simulink model "FBNREL_Ex05"  (Simulink 10.1)
settings: Solver=ode4  StartTime=0.0  StopTime=inf  FixedStep=dt  RelTol=1e-3  EnableMultiTasking=on
undefined symbols (not defined in the file or in its folder): Parameter
libraries: simulink x1
settings Model: Creator=ivohoutzager  LastModifiedBy=109813  ParamWorkspaceSource=ReferencedWorkspace
settings DataIOCC: LimitDataPoints=on  SaveOutput=off  SignalLogging=off  SaveTime=off
settings OptimizationCC: DefaultParameterBehavior=Inlined  ExpressionDepthLimit=2147483647
settings DebuggingCC: SolverPrmCheckMsg=warning  InheritedTsInSrcMsg=none  FcnCallInpInsideContextMsg=warning  AllowSymbolicDim=off  StateNameClashWarn=warning
settings RTWCC: Description=Bladed Style DLL  SystemTargetFile=discon_grt.tlc  TemplateMakefile=discon_vc_05.tmf  TargetLang=C++  RTWCompilerOptimization=on
settings RTWCC: CustomSource=|
  | Helpers.cpp
  | ExternalParameters.cpp
  | LegacyExternalControllerApi.cpp
settings CodeAppCC: MaxIdLength=63
settings GRTTargetCC: CombineOutputUpdateFcns=on  GRTInterface=off  UseToolchainInfoCompliant=off

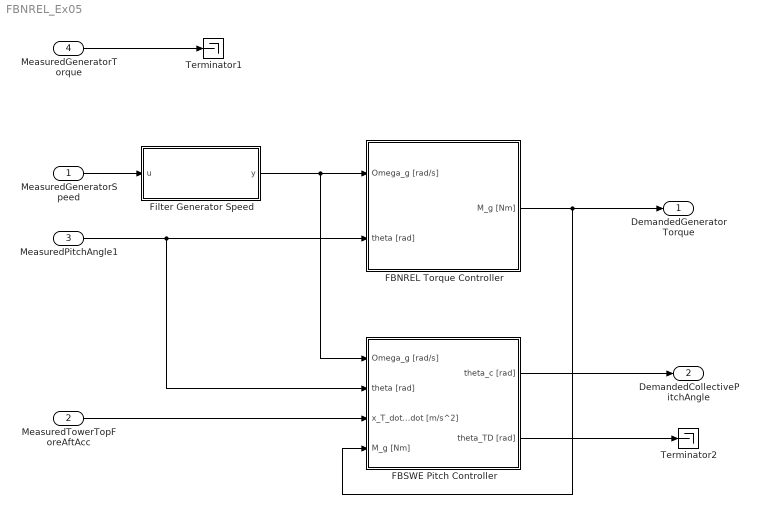
== system FBNREL_Ex05 ==
  MeasuredGeneratorSpeed : Inport  PortDimensions=1
  MeasuredTowerTopForeAftAcc : Inport  Port=2  PortDimensions=1
  MeasuredPitchAngle1 : Inport  Port=3  PortDimensions=1
  MeasuredGeneratorTorque : Inport  Port=4  PortDimensions=1
  FBNREL Torque Controller : Subsystem
  FBSWE Pitch Controller : Subsystem
  Filter Generator Speed : Subsystem
  Terminator1 : Terminator
  Terminator2 : Terminator
  DemandedGeneratorTorque : Outport  PortDimensions=1
  DemandedCollectivePitchAngle : Outport  Port=2  PortDimensions=1
  wires:
  MeasuredGeneratorTorque/1 -> Terminator1/1
  FBNREL Torque Controller/1(M_g [Nm]) -> FBSWE Pitch Controller/4(M_g [Nm]), DemandedGeneratorTorque/1
  MeasuredPitchAngle1/1 -> FBSWE Pitch Controller/2(theta [rad]), FBNREL Torque Controller/2(theta [rad])
  MeasuredGeneratorSpeed/1 -> Filter Generator Speed/1(u)
  Filter Generator Speed/1(y) -> FBSWE Pitch Controller/1(Omega_g [rad/s]), FBNREL Torque Controller/1(Omega_g [rad/s])
  FBSWE Pitch Controller/1(theta_c [rad]) -> DemandedCollectivePitchAngle/1
  FBSWE Pitch Controller/2(theta_TD [rad]) -> Terminator2/1
  MeasuredTowerTopForeAftAcc/1 -> FBSWE Pitch Controller/3(x_T_dotdot [m/s^2])

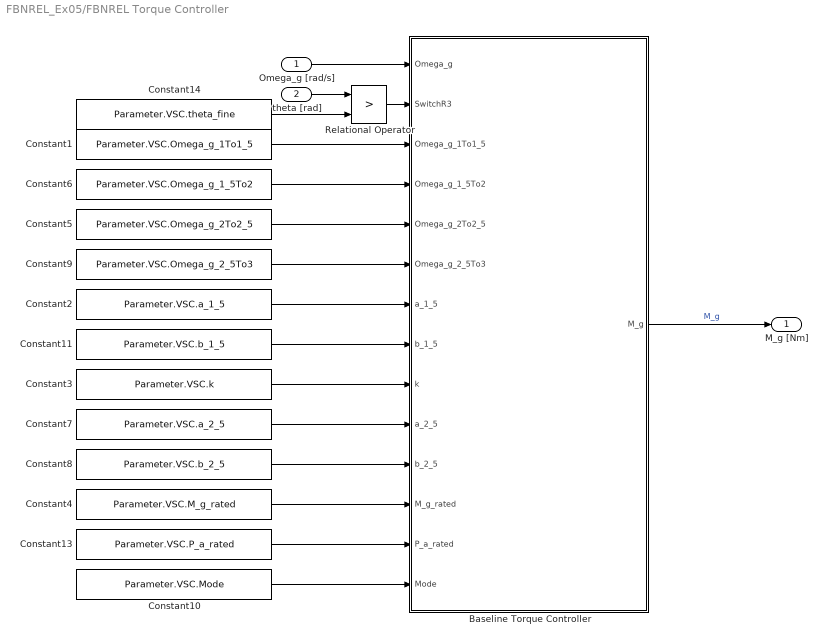
== system FBNREL_Ex05/FBNREL Torque Controller ==
  Omega_g [rad/s] : Inport
  theta [rad] : Inport  Port=2
  Baseline Torque Controller : MATLAB Function  TreatAsAtomicUnit=on
  Constant1 : Constant  Value=Parameter.VSC.Omega_g_1To1_5
  Constant10 : Constant  Value=Parameter.VSC.Mode
  Constant11 : Constant  Value=Parameter.VSC.b_1_5
  Constant13 : Constant  Value=Parameter.VSC.P_a_rated
  Constant14 : Constant  Value=Parameter.VSC.theta_fine
  Constant2 : Constant  Value=Parameter.VSC.a_1_5
  Constant3 : Constant  Value=Parameter.VSC.k
  Constant4 : Constant  Value=Parameter.VSC.M_g_rated
  Constant5 : Constant  Value=Parameter.VSC.Omega_g_2To2_5
  Constant6 : Constant  Value=Parameter.VSC.Omega_g_1_5To2
  Constant7 : Constant  Value=Parameter.VSC.a_2_5
  Constant8 : Constant  Value=Parameter.VSC.b_2_5
  Constant9 : Constant  Value=Parameter.VSC.Omega_g_2_5To3
  Relational Operator : RelationalOperator  Operator=>  OutDataTypeStr=boolean  RndMeth=Nearest
  M_g [Nm] : Outport
  wires:
  Constant13/1 -> Baseline Torque Controller/13(P_a_rated)
  Constant11/1 -> Baseline Torque Controller/8(b_1_5)
  Constant2/1 -> Baseline Torque Controller/7(a_1_5)
  Constant10/1 -> Baseline Torque Controller/14(Mode)
  Constant3/1 -> Baseline Torque Controller/9(k)
  Constant7/1 -> Baseline Torque Controller/10(a_2_5)
  Constant8/1 -> Baseline Torque Controller/11(b_2_5)
  Constant4/1 -> Baseline Torque Controller/12(M_g_rated)
  Constant9/1 -> Baseline Torque Controller/6(Omega_g_2_5To3)
  Constant6/1 -> Baseline Torque Controller/4(Omega_g_1_5To2)
  Constant5/1 -> Baseline Torque Controller/5(Omega_g_2To2_5)
  Constant1/1 -> Baseline Torque Controller/3(Omega_g_1To1_5)
  Baseline Torque Controller/1(M_g) -> M_g [Nm]/1  "M_g"
  Omega_g [rad/s]/1 -> Baseline Torque Controller/1(Omega_g)
  Constant14/1 -> Relational Operator/2
  theta [rad]/1 -> Relational Operator/1
  Relational Operator/1 -> Baseline Torque Controller/2(SwitchR3)

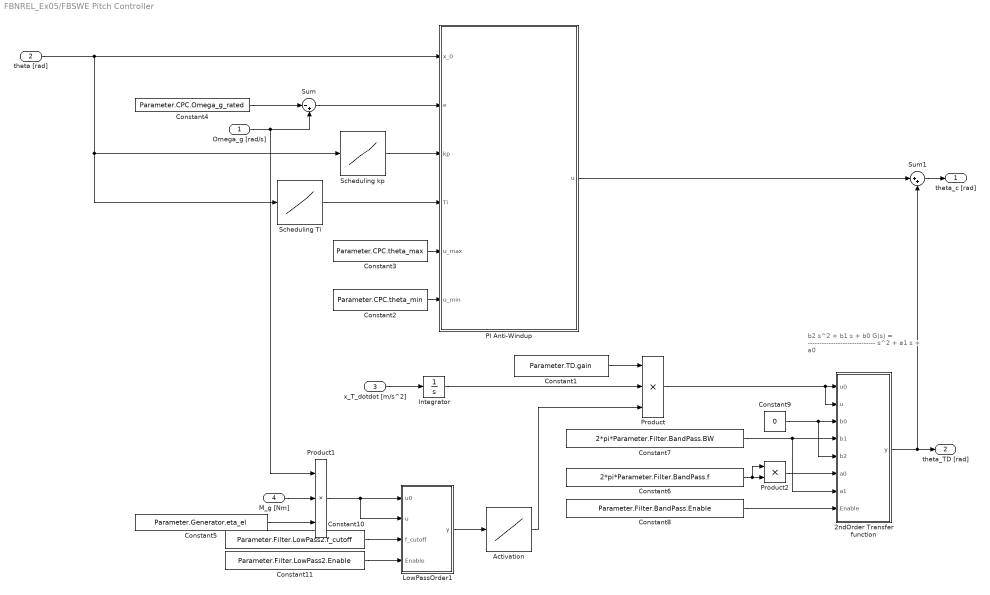
== system FBNREL_Ex05/FBSWE Pitch Controller ==
  note: b2 s^2 + b1 s + b0
      | G(s) = -----------------------------
      | s^2 + a1 s + a0
  Omega_g [rad/s] : Inport
  theta [rad] : Inport  Port=2
  x_T_dotdot [m/s^2] : Inport  Port=3
  M_g [Nm] : Inport  Port=4
  2ndOrder Transfer function : Subsystem
  Activation : Lookup_n-D  NumberOfTableDimensions=1  BreakpointsForDimension1=Parameter.TD.Power  IndexSearchMethod=Linear search  Table=Parameter.TD.Value  ExtrapMethod=Clip  UseLastTableValue=on  InternalRulePriority=Speed  RndMeth=Simplest  InputSameDT=on
  Constant1 : Constant  Value=Parameter.TD.gain
  Constant10 : Constant  Value=Parameter.Filter.LowPass2.f_cutoff
  Constant11 : Constant  Value=Parameter.Filter.LowPass2.Enable
  Constant2 : Constant  Value=Parameter.CPC.theta_min
  Constant3 : Constant  Value=Parameter.CPC.theta_max
  Constant4 : Constant  Value=Parameter.CPC.Omega_g_rated
  Constant5 : Constant  Value=Parameter.Generator.eta_el
  Constant6 : Constant  Value=2*pi*Parameter.Filter.BandPass.f
  Constant7 : Constant  Value=2*pi*Parameter.Filter.BandPass.BW
  Constant8 : Constant  Value=Parameter.Filter.BandPass.Enable
  Constant9 : Constant  Value=0
  Integrator : Integrator
  LowPassOrder1 : Subsystem
  PI Anti-Windup : Subsystem
  Product : Product  Inputs=3
  Product1 : Product  Inputs=***  RndMeth=Zero
  Product2 : Product  RndMeth=Zero
  Scheduling Ti : Lookup_n-D  NumberOfTableDimensions=1  BreakpointsForDimension1=Parameter.CPC.GS.theta  IndexSearchMethod=Linear search  Table=Parameter.CPC.GS.Ti  ExtrapMethod=Clip  UseLastTableValue=on  InternalRulePriority=Speed  RndMeth=Simplest  InputSameDT=on
  Scheduling kp : Lookup_n-D  NumberOfTableDimensions=1  BreakpointsForDimension1=Parameter.CPC.GS.theta  IndexSearchMethod=Linear search  Table=Parameter.CPC.GS.kp  ExtrapMethod=Clip  UseLastTableValue=on  InternalRulePriority=Speed  RndMeth=Simplest  InputSameDT=on
  Sum : Sum  Inputs=|-+
  Sum1 : Sum  Inputs=|++
  theta_c [rad] : Outport
  theta_TD [rad] : Outport  Port=2
  wires:
  Scheduling Ti/1 -> PI Anti-Windup/4(Ti)
  Scheduling kp/1 -> PI Anti-Windup/3(kp)
  theta [rad]/1 -> PI Anti-Windup/1(x_0), Scheduling kp/1, Scheduling Ti/1
  Omega_g [rad/s]/1 -> Product1/1, Sum/2
  Sum/1 -> PI Anti-Windup/2(e)
  Constant2/1 -> PI Anti-Windup/6(u_min)
  Constant3/1 -> PI Anti-Windup/5(u_max)
  Constant4/1 -> Sum/1
  PI Anti-Windup/1(u) -> Sum1/1
  Sum1/1 -> theta_c [rad]/1
  x_T_dotdot [m/s^2]/1 -> Integrator/1
  Integrator/1 -> Product/2
  Constant1/1 -> Product/1
  Activation/1 -> Product/3
  Product/1 -> 2ndOrder Transfer function/2(u), 2ndOrder Transfer function/1(u0)
  Constant8/1 -> 2ndOrder Transfer function/8(Enable)
  Product2/1 -> 2ndOrder Transfer function/6(a0)
  Constant6/1 -> Product2/1, Product2/2
  Constant7/1 -> 2ndOrder Transfer function/7(a1), 2ndOrder Transfer function/4(b1)
  Constant9/1 -> 2ndOrder Transfer function/5(b2), 2ndOrder Transfer function/3(b0)
  Product1/1 -> LowPassOrder1/2(u), LowPassOrder1/1(u0)
  Constant11/1 -> LowPassOrder1/4(Enable)
  Constant10/1 -> LowPassOrder1/3(f_cutoff)
  LowPassOrder1/1(y) -> Activation/1
  M_g [Nm]/1 -> Product1/2
  Constant5/1 -> Product1/3
  2ndOrder Transfer function/1(y) -> theta_TD [rad]/1, Sum1/2

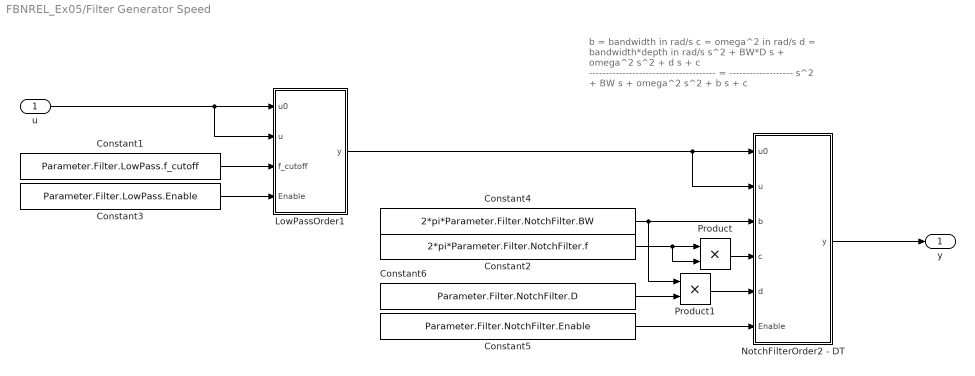
== system FBNREL_Ex05/Filter Generator Speed ==
  note: b = bandwidth in rad/s
      | c = omega^2 in rad/s
      | d = bandwidth*depth in rad/s
      |
      | s^2 + BW*D s + omega^2 s^2 + d s + c
      | -------------------------------------- = -------------------
      | s^2 + BW s + omega^2 s^2 + b s + c
  u : Inport
  Constant1 : Constant  Value=Parameter.Filter.LowPass.f_cutoff
  Constant2 : Constant  Value=2*pi*Parameter.Filter.NotchFilter.f
  Constant3 : Constant  Value=Parameter.Filter.LowPass.Enable
  Constant4 : Constant  Value=2*pi*Parameter.Filter.NotchFilter.BW
  Constant5 : Constant  Value=Parameter.Filter.NotchFilter.Enable
  Constant6 : Constant  Value=Parameter.Filter.NotchFilter.D
  LowPassOrder1 : Subsystem
  NotchFilterOrder2 - DT : Subsystem
  Product : Product  RndMeth=Zero
  Product1 : Product  RndMeth=Zero
  y : Outport
  wires:
  u/1 -> LowPassOrder1/2(u), LowPassOrder1/1(u0)
  Constant3/1 -> LowPassOrder1/4(Enable)
  Constant1/1 -> LowPassOrder1/3(f_cutoff)
  LowPassOrder1/1(y) -> NotchFilterOrder2 - DT/1(u0), NotchFilterOrder2 - DT/2(u)
  Constant5/1 -> NotchFilterOrder2 - DT/6(Enable)
  Product/1 -> NotchFilterOrder2 - DT/4(c)
  Constant2/1 -> Product/2, Product/1
  Constant4/1 -> NotchFilterOrder2 - DT/3(b), Product1/1
  Product1/1 -> NotchFilterOrder2 - DT/5(d)
  Constant6/1 -> Product1/2
  NotchFilterOrder2 - DT/1(y) -> y/1

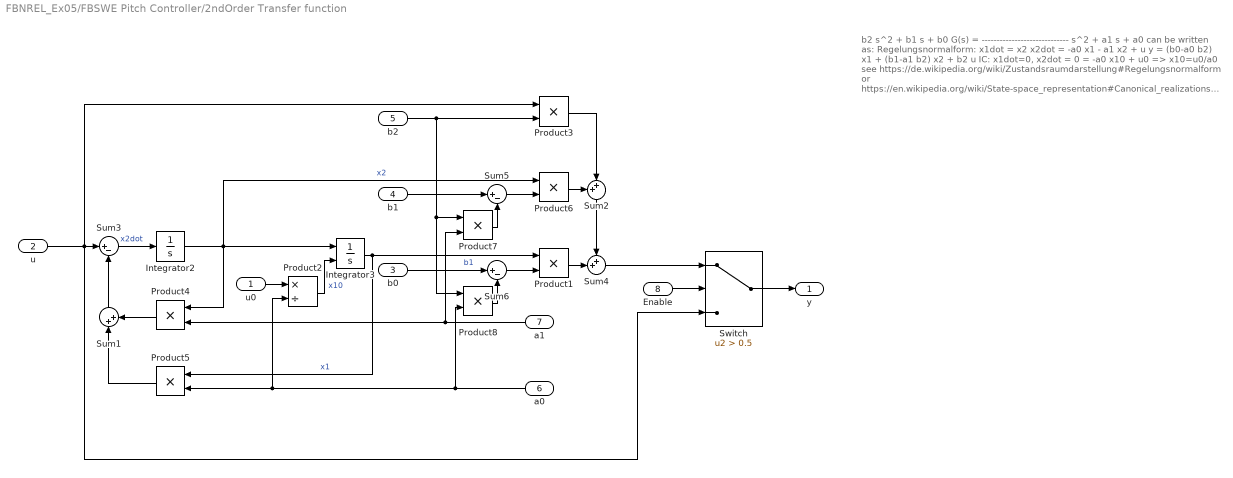
== system FBNREL_Ex05/FBSWE Pitch Controller/2ndOrder Transfer function ==
  note: b2 s^2 + b1 s + b0
      | G(s) = -----------------------------
      | s^2 + a1 s + a0
      |
      | can be written as:
      |
      | Regelungsnormalform:
      | x1dot = x2
      | x2dot = -a0 x1 - a1 x2 + u
      | y = (b0-a0 b2) x1 + (b1-a1 b2) x2 + b2 u
      |
      | IC: x1dot=0, x2dot = 0 = -a0 x10 + u0 => x10=u0/a0
      |
      | see https://de.wikipedia.org/wiki/Zustandsraumdarstellung#Regelungsnormalform
      | or
      | https://en.wikipedia.org/wiki/State-space_representation#Canonical_realizations
      |
      | Advantage:
      | - IC can be set
      | - coefficients can be changed online
  u0 : Inport
  u : Inport  Port=2
  b0 : Inport  Port=3
  b1 : Inport  Port=4
  b2 : Inport  Port=5
  a0 : Inport  Port=6
  a1 : Inport  Port=7
  Enable : Inport  Port=8
  Integrator2 : Integrator
  Integrator3 : Integrator  InitialConditionSource=external
  Product{1,3..8} (7 alike) : Product  RndMeth=Zero
  Product2 : Product  Inputs=*/  RndMeth=Zero
  Sum1 : Sum  Inputs=|++
  Sum2 : Sum  Inputs=++|
  Sum3 : Sum  Inputs=|+-
  Sum4 : Sum  Inputs=++|
  Sum5 : Sum  Inputs=|+-
  Sum6 : Sum  Inputs=|+-
  Switch : Switch  Criteria=u2 > Threshold  Threshold=0.5
  y : Outport
  wires:
  Switch/1 -> y/1
  Enable/1 -> Switch/2
  Integrator2/1 -> Integrator3/1, Product6/1, Product4/1  "x2"
  Integrator3/1 -> Product1/1, Product5/1  "x1"
  Sum3/1 -> Integrator2/1  "x2dot"
  u/1 -> Product3/1, Sum3/1, Switch/3
  Sum4/1 -> Switch/1
  Product1/1 -> Sum4/2
  Product6/1 -> Sum2/1
  Sum2/1 -> Sum4/1
  Sum1/1 -> Sum3/2
  Product4/1 -> Sum1/2
  Product5/1 -> Sum1/1
  a0/1 -> Product8/2, Product2/2, Product5/2
  a1/1 -> Product7/2, Product4/2
  b2/1 -> Product8/1, Product7/1, Product3/2
  Product3/1 -> Sum2/2
  Sum5/1 -> Product6/2
  b1/1 -> Sum5/1
  Product7/1 -> Sum5/2
  Sum6/1 -> Product1/2
  b0/1 -> Sum6/1  "b1"
  Product8/1 -> Sum6/2
  Product2/1 -> Integrator3/2  "x10"
  u0/1 -> Product2/1

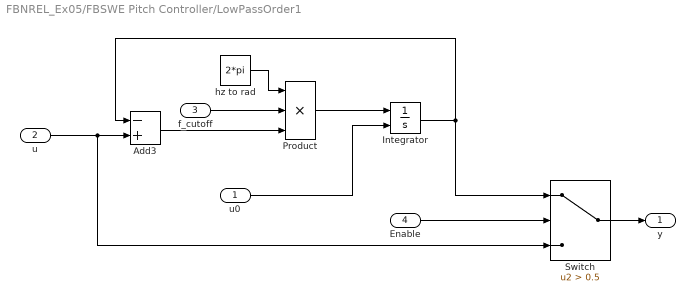
== system FBNREL_Ex05/FBSWE Pitch Controller/LowPassOrder1 ==
  u0 : Inport
  u : Inport  Port=2
  f_cutoff : Inport  Port=3
  Enable : Inport  Port=4
  Add3 : Sum  Inputs=-+
  Integrator : Integrator  InitialConditionSource=external
  Product : Product  Inputs=3  RndMeth=Zero
  Switch : Switch  Criteria=u2 > Threshold  Threshold=0.5
  hz to rad : Constant  Value=2*pi
  y : Outport
  wires:
  u0/1 -> Integrator/2
  Switch/1 -> y/1
  Enable/1 -> Switch/2
  u/1 -> Add3/2, Switch/3
  Integrator/1 -> Switch/1, Add3/1
  Product/1 -> Integrator/1
  Add3/1 -> Product/3
  f_cutoff/1 -> Product/2
  hz to rad/1 -> Product/1

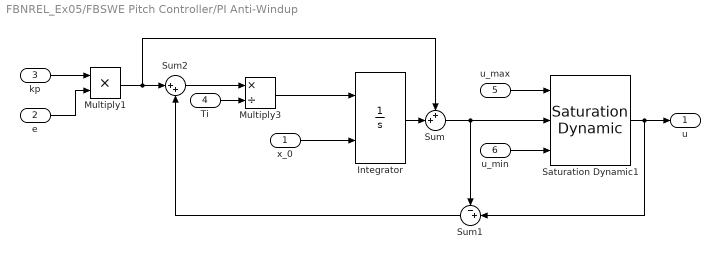
== system FBNREL_Ex05/FBSWE Pitch Controller/PI Anti-Windup ==
  x_0 : Inport
  e : Inport  Port=2
  kp : Inport  Port=3
  Ti : Inport  Port=4
  u_max : Inport  Port=5
  u_min : Inport  Port=6
  Integrator : Integrator  InitialConditionSource=external
  Multiply1 : Product  Inputs=**
  Multiply3 : Product  Inputs=*/
  Saturation Dynamic1 : simulink/Discontinuities/Saturation Dynamic  OutMin=[]  OutMax=[]  OutDataTypeStr=Inherit: Same as second input  OutDataType=fixdt(1, 16)  OutScaling=2^-10  DoSatur=off
  Sum : Sum  Inputs=++|
  Sum1 : Sum  Inputs=-+|
  Sum2 : Sum  Inputs=|++
  u : Outport
  wires:
  Saturation Dynamic1/1 -> u/1, Sum1/2
  Integrator/1 -> Sum/2
  kp/1 -> Multiply1/1
  e/1 -> Multiply1/2
  Ti/1 -> Multiply3/2
  Sum1/1 -> Sum2/2
  Multiply1/1 -> Sum/1, Sum2/1
  Sum2/1 -> Multiply3/1
  x_0/1 -> Integrator/2
  Multiply3/1 -> Integrator/1
  u_min/1 -> Saturation Dynamic1/3
  Sum/1 -> Saturation Dynamic1/2, Sum1/1
  u_max/1 -> Saturation Dynamic1/1

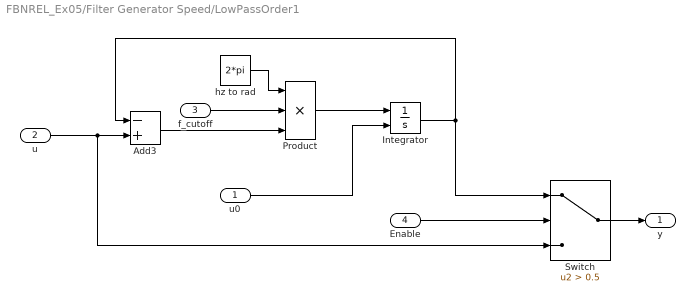
== system FBNREL_Ex05/Filter Generator Speed/LowPassOrder1 ==
  u0 : Inport
  u : Inport  Port=2
  f_cutoff : Inport  Port=3
  Enable : Inport  Port=4
  Add3 : Sum  Inputs=-+
  Integrator : Integrator  InitialConditionSource=external
  Product : Product  Inputs=3  RndMeth=Zero
  Switch : Switch  Criteria=u2 > Threshold  Threshold=0.5
  hz to rad : Constant  Value=2*pi
  y : Outport
  wires:
  u0/1 -> Integrator/2
  Switch/1 -> y/1
  Enable/1 -> Switch/2
  u/1 -> Add3/2, Switch/3
  Integrator/1 -> Switch/1, Add3/1
  Product/1 -> Integrator/1
  Add3/1 -> Product/3
  f_cutoff/1 -> Product/2
  hz to rad/1 -> Product/1

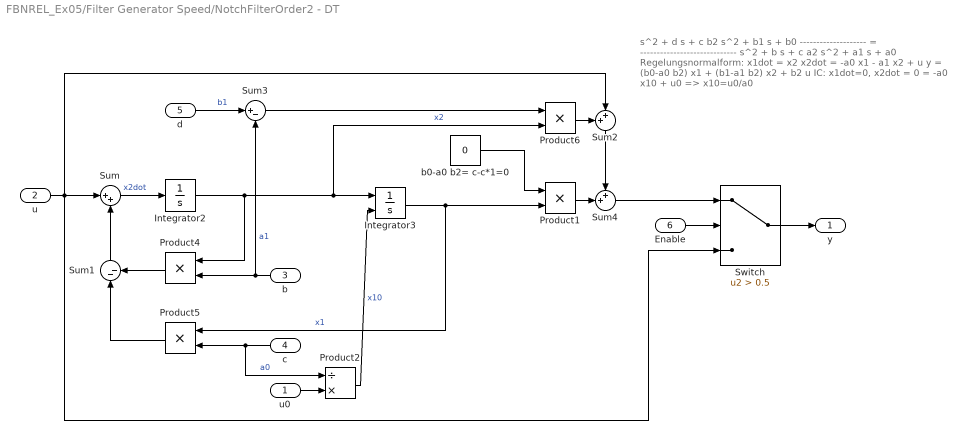
== system FBNREL_Ex05/Filter Generator Speed/NotchFilterOrder2 - DT ==
  note: s^2 + d s + c b2 s^2 + b1 s + b0
      | -------------------- = -----------------------------
      | s^2 + b s + c a2 s^2 + a1 s + a0
      |
      | Regelungsnormalform:
      | x1dot = x2
      | x2dot = -a0 x1 - a1 x2 + u
      | y = (b0-a0 b2) x1 + (b1-a1 b2) x2 + b2 u
      |
      | IC: x1dot=0, x2dot = 0 = -a0 x10 + u0 => x10=u0/a0
  u0 : Inport
  u : Inport  Port=2
  b : Inport  Port=3
  c : Inport  Port=4
  d : Inport  Port=5
  Enable : Inport  Port=6
  Integrator2 : Integrator
  Integrator3 : Integrator  InitialConditionSource=external
  Product{1,4..6} (4 alike) : Product  RndMeth=Zero
  Product2 : Product  Inputs=/*  RndMeth=Zero
  Sum : Sum  Inputs=|++
  Sum1 : Sum  Inputs=|--
  Sum2 : Sum  Inputs=++|
  Sum3 : Sum  Inputs=|+-
  Sum4 : Sum  Inputs=++|
  Switch : Switch  Criteria=u2 > Threshold  Threshold=0.5
  b0-a0 b2= c-c*1=0 : Constant  Value=0
  y : Outport
  wires:
  b0-a0 b2= c-c*1=0/1 -> Product1/1
  u0/1 -> Product2/2
  Sum2/1 -> Sum4/1
  Sum3/1 -> Product6/1
  Product6/1 -> Sum2/1
  Product1/1 -> Sum4/2
  Sum4/1 -> Switch/1
  c/1 -> Product5/2, Product2/1  "a0"
  b/1 -> Sum3/2, Product4/2  "a1"
  Product2/1 -> Integrator3/2  "x10"
  d/1 -> Sum3/1  "b1"
  u/1 -> Sum/1, Switch/3, Sum2/2
  Product5/1 -> Sum1/1
  Product4/1 -> Sum1/2
  Sum1/1 -> Sum/2
  Sum/1 -> Integrator2/1  "x2dot"
  Integrator3/1 -> Product1/2, Product5/1  "x1"
  Integrator2/1 -> Product4/1, Integrator3/1, Product6/2  "x2"
  Enable/1 -> Switch/2
  Switch/1 -> y/1

== matlab function FBNREL Torque Controller/Baseline Torque Controller ==
  settings: fimath=|
      | fimath(...
      | 'RoundMode', 'floor',...
      | 'OverflowMode', 'wrap',...
      | 'ProductMode', 'KeepLSB', 'ProductWordLength', 32,...
      | 'SumMode', 'KeepLSB', 'SumWordLength', 32,...
      | 'CastBeforeSum', false)
  data: Omega_g input double; SwitchR3 input double; Omega_g_1To1_5 input double; Omega_g_1_5To2 input double; Omega_g_2To2_5 input double; Omega_g_2_5To3 input double; a_1_5 input double; b_1_5 input double; k input double; a_2_5 input double; b_2_5 input double; M_g output double; M_g_rated input double; P_a_rated input double; Mode input double
function M_g = BaselineVSControl(Omega_g,SwitchR3,...  	% signals
    Omega_g_1To1_5,Omega_g_1_5To2,...
    Omega_g_2To2_5,Omega_g_2_5To3,...                   % region limits
    a_1_5,b_1_5,...                                    	% Region 1.5 parameters
    k,...                                             	% Region   2 parameters
    a_2_5,b_2_5,...                                    	% Region 2.5 parameters
    M_g_rated,P_a_rated,Mode)                        	% Region   3 parameters

if  Mode == 1                                         	% Power constant
    M_g_3 = P_a_rated/Omega_g;
else                                                    % Torque constant
    M_g_3 = M_g_rated;
end

if      Omega_g_2_5To3  <   Omega_g                     % Region 3
    M_g     = M_g_3;

elseif  Omega_g_2To2_5  <   Omega_g                     % Region 2.5
    M_g_2_5 = a_2_5 * Omega_g + b_2_5;
    M_g     = SwitchR3*M_g_3+(1-SwitchR3)*M_g_2_5;

elseif  Omega_g_1_5To2  <   Omega_g                     % Region 2
    M_g_2   = k * Omega_g^2;
    M_g     = SwitchR3*M_g_3+(1-SwitchR3)*M_g_2;  
    
elseif  Omega_g_1To1_5  <   Omega_g                     % Region 1.5
    M_g = a_1_5 * Omega_g + b_1_5;

else                                                    % Region 1 
    M_g = 0;    
end
